simulink model "asghb"  (R2016a)
settings: Solver=VariableStepAuto  StartTime=0.0  StopTime=500  RelTol=1e-3
values from neighbouring files (symbols this model uses):
  Ag = 0.8    [Valori.m]
  Dg1 = 40    [Valori.m]
  Dg2 = 60    [Valori.m]
  Dg3 = 80    [Valori.m]
  Gb = 80    [Valori.m]
  K1 = 55.55    [Valori.m]
  K2 = 1260000    [Valori.m]
  K3 = 132.312    [Valori.m]
  n = 0.109    [Valori.m]
  p1 = 0.029    [Valori.m]
  p2 = 0.029    [Valori.m]
  p3 = 0.00000783    (= 7.83e-06)    [Valori.m]
  tgmax = 40    [Valori.m]
  V = 120    [Valori.m]
settings Model: Creator=carme  LastModifiedBy=carme

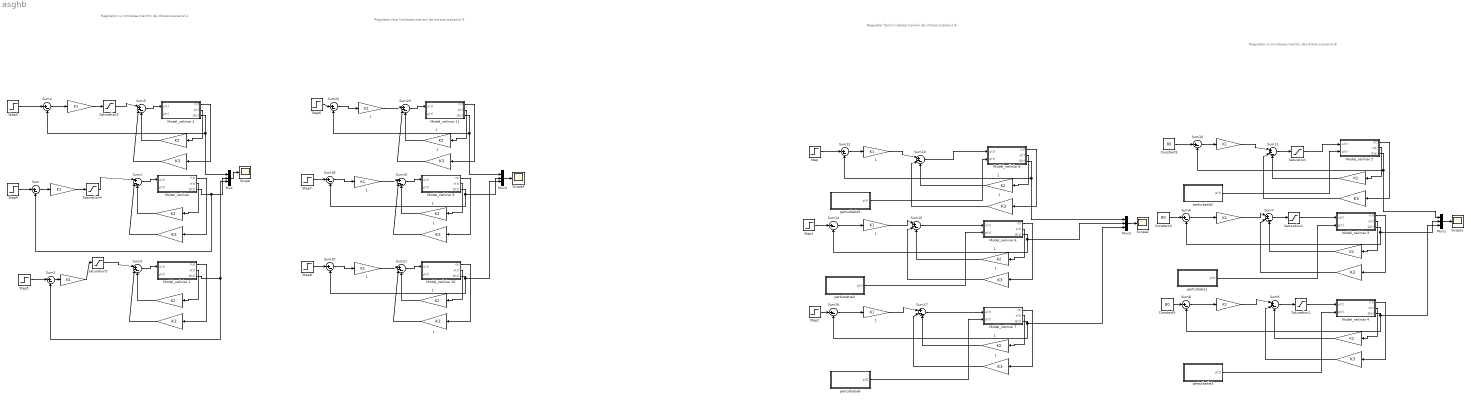
== system asghb ==
  note: Regulator cu limitarea marimii de intrare scenariul A
  note: Regulator cu limitarea marimii de intrare scenariul B
  note: Regulator fara limitarea marimii de intrare scenariul B
  note: Regulator fara limitarea marimii de intrare scenariul A
   {,,1,1} (4 alike) : Gain  Gain=K1
  "   " : Gain  Gain=K3
  "      " : Gain  Gain=K3
  "       " : Gain  Gain=K2
  "        " : Gain  Gain=K2
  "          " : Gain  Gain=K3
  "              " : Gain  Gain=K2
  "               " : Gain  Gain=K1
  " " : Gain  Gain=K2
  " 1" : Gain  Gain=K2
  "                                  " : Gain  Gain=K3
  "                                        " : Gain  Gain=K1
  "                                           " : Gain  Gain=K1
  "                                            " : Gain  Gain=K3
  "                                                        " : Gain  Gain=K1
  "                                                             " : Gain  Gain=K3
  "                                                                     " : Gain  Gain=K2
  "                                                                                           " : Gain  Gain=K2
  "                                                                                           1" : Gain  Gain=K2
  "                                                                     1" : Gain  Gain=K2
  "                                                             1" : Gain  Gain=K3
  "                                                        1" : Gain  Gain=K1
  "                                            1" : Gain  Gain=K3
  "                                           1" : Gain  Gain=K1
  "                                        1" : Gain  Gain=K1
  "                                  1" : Gain  Gain=K3
  "               1" : Gain  Gain=K1
  "              1" : Gain  Gain=K2
  "          1" : Gain  Gain=K3
  "        1" : Gain  Gain=K2
  "       1" : Gain  Gain=K2
  "      1" : Gain  Gain=K3
  "   1" : Gain  Gain=K3
  Constant3 : Constant  Value=80
  Constant4 : Constant  Value=80
  Constant5 : Constant  Value=80
  "Model_neliniar " : Subsystem
  Model_neliniar 1 : Subsystem
  Model_neliniar 10 : Subsystem
  Model_neliniar 11 : Subsystem
  Model_neliniar 2 : Subsystem
  Model_neliniar 3 : Subsystem
  Model_neliniar 4 : Subsystem
  Model_neliniar 5 : Subsystem
  Model_neliniar 6 : Subsystem
  Model_neliniar 7 : Subsystem
  Model_neliniar 8 : Subsystem
  Model_neliniar 9 : Subsystem
  Mux{,1..3} (4 alike) : Mux  Inputs=3
  Saturation{,1..5} (6 alike) : Saturate
  Scope{,1..3} (4 alike) : Scope
  Step{,1..8} (9 alike) : Step  SampleTime=0
  Sum{,2,4,6,8,10,12,14,16,18,20,22} (12 alike) : Sum  Inputs=|+-
  Sum{1,3,5,7,9,11,13,15,17,19,21,23} (12 alike) : Sum  Inputs=|+--
  perturbatie1 : Subsystem
  perturbatie2 : Subsystem
  perturbatie3 : Subsystem
  perturbatie4 : Subsystem
  perturbatie5 : Subsystem
  perturbatie6 : Subsystem
  wires:
  Sum1/1 -> "Model_neliniar "/1(u(t))
  "Model_neliniar "/3(G(t)) -> Mux/2, Sum/2
  "Model_neliniar "/1(i(t)) -> "                                  "/1
  "Model_neliniar "/2(x(t)) -> "                                                                     "/1
  "                                  "/1 -> Sum1/2
  "                                                                     "/1 -> Sum1/3
  Step4/1 -> Sum/1
  Sum/1 -> "                                                        "/1
  Sum3/1 -> Model_neliniar 1/1(u(t))
  Model_neliniar 1/3(G(t)) -> Mux/3, Sum2/2
  Model_neliniar 1/1(i(t)) -> "                                                             "/1
  Model_neliniar 1/2(x(t)) -> "                                                                                           "/1
  "                                                             "/1 -> Sum3/2
  "                                                                                           "/1 -> Sum3/3
  Step5/1 -> Sum2/1
  Sum2/1 -> "                                        "/1
  Sum5/1 -> Model_neliniar 2/1(u(t))
  Model_neliniar 2/3(G(t)) -> Mux/1, Sum4/2
  Model_neliniar 2/1(i(t)) -> "                                            "/1
  Model_neliniar 2/2(x(t)) -> "              "/1
  "                                            "/1 -> Sum5/2
  "              "/1 -> Sum5/3
  Step3/1 -> Sum4/1
  Sum4/1 -> " "/1
  Mux/1 -> Scope/1
  "               "/1 -> Sum7/1
  Model_neliniar 3/3(G(t)) -> Mux1/2, Sum6/2
  Model_neliniar 3/1(i(t)) -> "      "/1
  Model_neliniar 3/2(x(t)) -> "        "/1
  "      "/1 -> Sum7/2
  "        "/1 -> Sum7/3
  Constant4/1 -> Sum6/1
  Sum6/1 -> "               "/1
  "                                           "/1 -> Sum9/1
  Model_neliniar 4/3(G(t)) -> Mux1/3, Sum8/2
  Model_neliniar 4/1(i(t)) -> "   "/1
  Model_neliniar 4/2(x(t)) -> "       "/1
  "   "/1 -> Sum9/2
  "       "/1 -> Sum9/3
  Constant5/1 -> Sum8/1
  Sum8/1 -> "                                           "/1
  " "/1 -> Sum11/1
  Model_neliniar 5/3(G(t)) -> Mux1/1, Sum10/2
  Model_neliniar 5/1(i(t)) -> "          "/1
  Model_neliniar 5/2(x(t)) -> " "/1
  "          "/1 -> Sum11/2
  " "/1 -> Sum11/3
  Constant3/1 -> Sum10/1
  Sum10/1 -> " "/1
  Mux1/1 -> Scope1/1
  Sum11/1 -> Saturation/1
  Saturation/1 -> Model_neliniar 5/1(u(t))
  Sum7/1 -> Saturation1/1
  Saturation1/1 -> Model_neliniar 3/1(u(t))
  Sum9/1 -> Saturation2/1
  Saturation2/1 -> Model_neliniar 4/1(u(t))
  perturbatie2/1(p(t)) -> Model_neliniar 5/2(p(t))
  perturbatie1/1(p(t)) -> Model_neliniar 3/2(p(t))
  perturbatie3/1(p(t)) -> Model_neliniar 4/2(p(t))
  "               1"/1 -> Sum15/1
  Model_neliniar 6/3(G(t)) -> Mux2/2, Sum14/2
  Model_neliniar 6/1(i(t)) -> "      1"/1
  Model_neliniar 6/2(x(t)) -> "        1"/1
  "      1"/1 -> Sum15/2
  "        1"/1 -> Sum15/3
  Step1/1 -> Sum14/1
  Sum14/1 -> "               1"/1
  "                                           1"/1 -> Sum17/1
  Model_neliniar 7/3(G(t)) -> Mux2/3, Sum16/2
  Model_neliniar 7/1(i(t)) -> "   1"/1
  Model_neliniar 7/2(x(t)) -> "       1"/1
  "   1"/1 -> Sum17/2
  "       1"/1 -> Sum17/3
  Step2/1 -> Sum16/1
  Sum16/1 -> "                                           1"/1
  " 1"/1 -> Sum13/1
  Model_neliniar 8/3(G(t)) -> Mux2/1, Sum12/2
  Model_neliniar 8/1(i(t)) -> "          1"/1
  Model_neliniar 8/2(x(t)) -> " 1"/1
  "          1"/1 -> Sum13/2
  " 1"/1 -> Sum13/3
  Step/1 -> Sum12/1
  Sum12/1 -> " 1"/1
  Mux2/1 -> Scope2/1
  Sum13/1 -> Model_neliniar 8/1(u(t))
  Sum15/1 -> Model_neliniar 6/1(u(t))
  Sum17/1 -> Model_neliniar 7/1(u(t))
  perturbatie5/1(p(t)) -> Model_neliniar 8/2(p(t))
  perturbatie4/1(p(t)) -> Model_neliniar 6/2(p(t))
  perturbatie6/1(p(t)) -> Model_neliniar 7/2(p(t))
  "                                                        1"/1 -> Sum19/1
  Sum19/1 -> Model_neliniar 9/1(u(t))
  Model_neliniar 9/3(G(t)) -> Mux3/2, Sum18/2
  Model_neliniar 9/1(i(t)) -> "                                  1"/1
  Model_neliniar 9/2(x(t)) -> "                                                                     1"/1
  "                                  1"/1 -> Sum19/2
  "                                                                     1"/1 -> Sum19/3
  Step7/1 -> Sum18/1
  Sum18/1 -> "                                                        1"/1
  "                                        1"/1 -> Sum21/1
  Sum21/1 -> Model_neliniar 10/1(u(t))
  Model_neliniar 10/3(G(t)) -> Mux3/3, Sum20/2
  Model_neliniar 10/1(i(t)) -> "                                                             1"/1
  Model_neliniar 10/2(x(t)) -> "                                                                                           1"/1
  "                                                             1"/1 -> Sum21/2
  "                                                                                           1"/1 -> Sum21/3
  Step8/1 -> Sum20/1
  Sum20/1 -> "                                        1"/1
  " 1"/1 -> Sum23/1
  Sum23/1 -> Model_neliniar 11/1(u(t))
  Model_neliniar 11/3(G(t)) -> Mux3/1, Sum22/2
  Model_neliniar 11/1(i(t)) -> "                                            1"/1
  Model_neliniar 11/2(x(t)) -> "              1"/1
  "                                            1"/1 -> Sum23/2
  "              1"/1 -> Sum23/3
  Step6/1 -> Sum22/1
  Sum22/1 -> " 1"/1
  Mux3/1 -> Scope3/1
  " "/1 -> Saturation3/1
  Saturation3/1 -> Sum5/1
  "                                                        "/1 -> Saturation4/1
  Saturation4/1 -> Sum1/1
  "                                        "/1 -> Saturation5/1
  Saturation5/1 -> Sum3/1

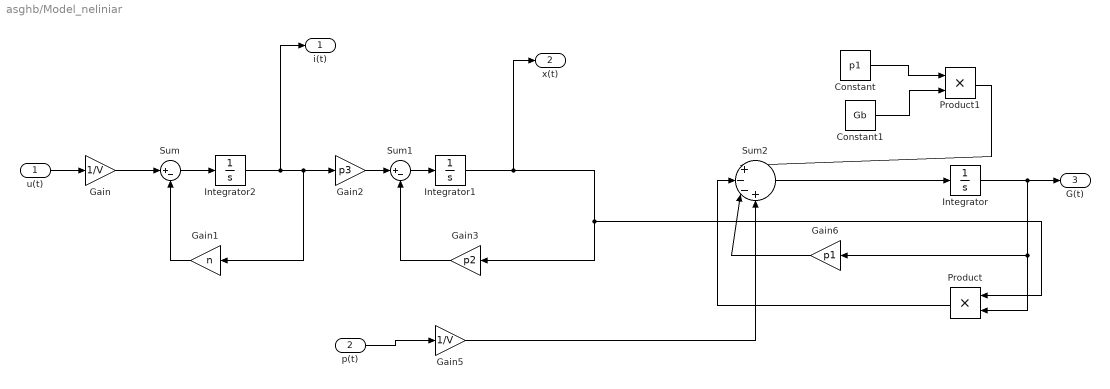
== system asghb/Model_neliniar  ==
  u(t) : Inport
  p(t) : Inport  Port=2
  Constant : Constant  Value=p1
  Constant1 : Constant  Value=Gb
  Gain : Gain  Gain=1/V
  Gain1 : Gain  Gain=n
  Gain2 : Gain  Gain=p3
  Gain3 : Gain  Gain=p2
  Gain5 : Gain  Gain=1/V
  Gain6 : Gain  Gain=p1
  Integrator : Integrator  InitialCondition=200
  Integrator1 : Integrator
  Integrator2 : Integrator
  Product : Product
  Product1 : Product
  Sum : Sum  Inputs=|+-
  Sum1 : Sum  Inputs=|+-
  Sum2 : Sum  Inputs=|+--+
  i(t) : Outport
  x(t) : Outport  Port=2
  G(t) : Outport  Port=3
  wires:
  u(t)/1 -> Gain/1
  Gain/1 -> Sum/1
  Sum/1 -> Integrator2/1
  Integrator2/1 -> i(t)/1, Gain1/1, Gain2/1
  Gain2/1 -> Sum1/1
  Sum1/1 -> Integrator1/1
  Gain1/1 -> Sum/2
  Gain3/1 -> Sum1/2
  Integrator1/1 -> x(t)/1, Product/1, Gain3/1
  p(t)/1 -> Gain5/1
  Gain5/1 -> Sum2/4
  Integrator/1 -> Product/2, Gain6/1, G(t)/1
  Gain6/1 -> Sum2/3
  Constant/1 -> Product1/1
  Constant1/1 -> Product1/2
  Product1/1 -> Sum2/1
  Product/1 -> Sum2/2
  Sum2/1 -> Integrator/1

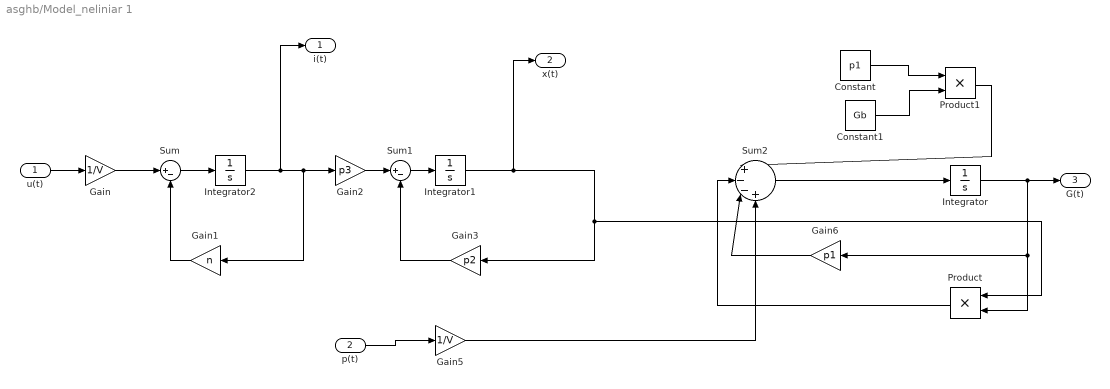
== system asghb/Model_neliniar 1 ==
  u(t) : Inport
  p(t) : Inport  Port=2
  Constant : Constant  Value=p1
  Constant1 : Constant  Value=Gb
  Gain : Gain  Gain=1/V
  Gain1 : Gain  Gain=n
  Gain2 : Gain  Gain=p3
  Gain3 : Gain  Gain=p2
  Gain5 : Gain  Gain=1/V
  Gain6 : Gain  Gain=p1
  Integrator : Integrator  InitialCondition=300
  Integrator1 : Integrator
  Integrator2 : Integrator
  Product : Product
  Product1 : Product
  Sum : Sum  Inputs=|+-
  Sum1 : Sum  Inputs=|+-
  Sum2 : Sum  Inputs=|+--+
  i(t) : Outport
  x(t) : Outport  Port=2
  G(t) : Outport  Port=3
  wires:
  u(t)/1 -> Gain/1
  Gain/1 -> Sum/1
  Sum/1 -> Integrator2/1
  Integrator2/1 -> i(t)/1, Gain1/1, Gain2/1
  Gain2/1 -> Sum1/1
  Sum1/1 -> Integrator1/1
  Gain1/1 -> Sum/2
  Gain3/1 -> Sum1/2
  Integrator1/1 -> x(t)/1, Product/1, Gain3/1
  p(t)/1 -> Gain5/1
  Gain5/1 -> Sum2/4
  Integrator/1 -> Product/2, Gain6/1, G(t)/1
  Gain6/1 -> Sum2/3
  Constant/1 -> Product1/1
  Constant1/1 -> Product1/2
  Product1/1 -> Sum2/1
  Product/1 -> Sum2/2
  Sum2/1 -> Integrator/1

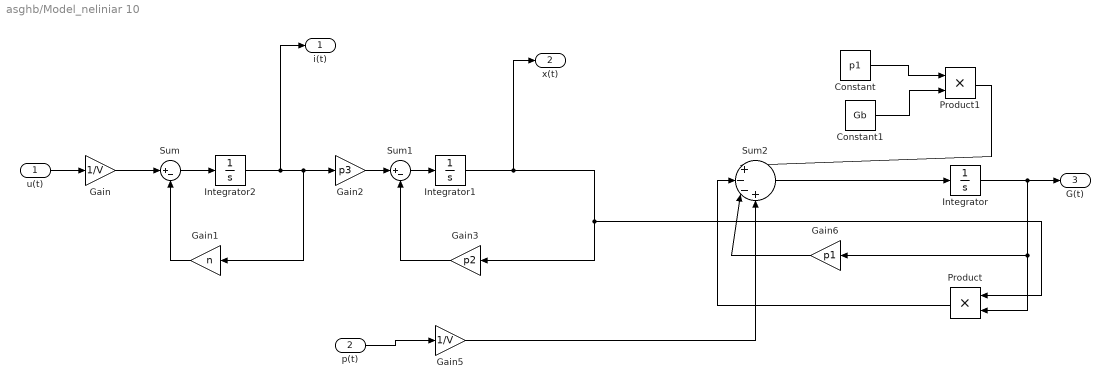
== system asghb/Model_neliniar 10 ==
  u(t) : Inport
  p(t) : Inport  Port=2
  Constant : Constant  Value=p1
  Constant1 : Constant  Value=Gb
  Gain : Gain  Gain=1/V
  Gain1 : Gain  Gain=n
  Gain2 : Gain  Gain=p3
  Gain3 : Gain  Gain=p2
  Gain5 : Gain  Gain=1/V
  Gain6 : Gain  Gain=p1
  Integrator : Integrator  InitialCondition=300
  Integrator1 : Integrator
  Integrator2 : Integrator
  Product : Product
  Product1 : Product
  Sum : Sum  Inputs=|+-
  Sum1 : Sum  Inputs=|+-
  Sum2 : Sum  Inputs=|+--+
  i(t) : Outport
  x(t) : Outport  Port=2
  G(t) : Outport  Port=3
  wires:
  u(t)/1 -> Gain/1
  Gain/1 -> Sum/1
  Sum/1 -> Integrator2/1
  Integrator2/1 -> i(t)/1, Gain1/1, Gain2/1
  Gain2/1 -> Sum1/1
  Sum1/1 -> Integrator1/1
  Gain1/1 -> Sum/2
  Gain3/1 -> Sum1/2
  Integrator1/1 -> x(t)/1, Product/1, Gain3/1
  p(t)/1 -> Gain5/1
  Gain5/1 -> Sum2/4
  Integrator/1 -> Product/2, Gain6/1, G(t)/1
  Gain6/1 -> Sum2/3
  Constant/1 -> Product1/1
  Constant1/1 -> Product1/2
  Product1/1 -> Sum2/1
  Product/1 -> Sum2/2
  Sum2/1 -> Integrator/1

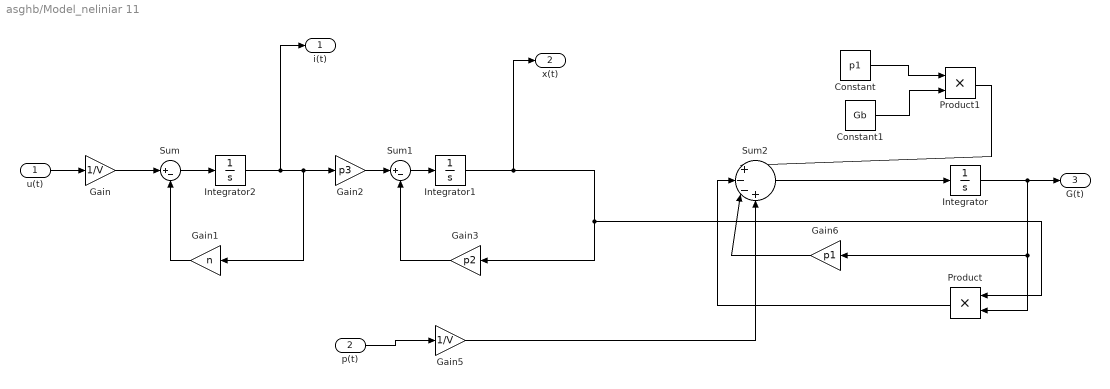
== system asghb/Model_neliniar 11 ==
  u(t) : Inport
  p(t) : Inport  Port=2
  Constant : Constant  Value=p1
  Constant1 : Constant  Value=Gb
  Gain : Gain  Gain=1/V
  Gain1 : Gain  Gain=n
  Gain2 : Gain  Gain=p3
  Gain3 : Gain  Gain=p2
  Gain5 : Gain  Gain=1/V
  Gain6 : Gain  Gain=p1
  Integrator : Integrator  InitialCondition=120
  Integrator1 : Integrator
  Integrator2 : Integrator
  Product : Product
  Product1 : Product
  Sum : Sum  Inputs=|+-
  Sum1 : Sum  Inputs=|+-
  Sum2 : Sum  Inputs=|+--+
  i(t) : Outport
  x(t) : Outport  Port=2
  G(t) : Outport  Port=3
  wires:
  u(t)/1 -> Gain/1
  Gain/1 -> Sum/1
  Sum/1 -> Integrator2/1
  Integrator2/1 -> i(t)/1, Gain1/1, Gain2/1
  Gain2/1 -> Sum1/1
  Sum1/1 -> Integrator1/1
  Gain1/1 -> Sum/2
  Gain3/1 -> Sum1/2
  Integrator1/1 -> x(t)/1, Product/1, Gain3/1
  p(t)/1 -> Gain5/1
  Gain5/1 -> Sum2/4
  Integrator/1 -> Product/2, Gain6/1, G(t)/1
  Gain6/1 -> Sum2/3
  Constant/1 -> Product1/1
  Constant1/1 -> Product1/2
  Product1/1 -> Sum2/1
  Product/1 -> Sum2/2
  Sum2/1 -> Integrator/1

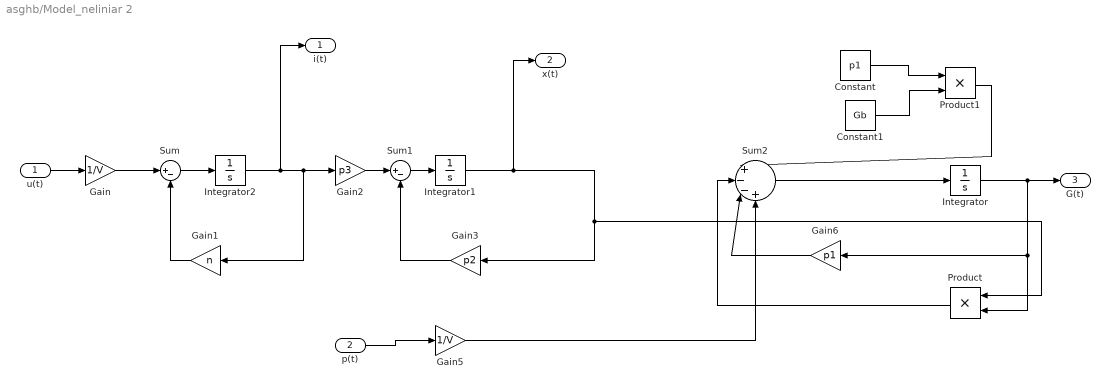
== system asghb/Model_neliniar 2 ==
  u(t) : Inport
  p(t) : Inport  Port=2
  Constant : Constant  Value=p1
  Constant1 : Constant  Value=Gb
  Gain : Gain  Gain=1/V
  Gain1 : Gain  Gain=n
  Gain2 : Gain  Gain=p3
  Gain3 : Gain  Gain=p2
  Gain5 : Gain  Gain=1/V
  Gain6 : Gain  Gain=p1
  Integrator : Integrator  InitialCondition=120
  Integrator1 : Integrator
  Integrator2 : Integrator
  Product : Product
  Product1 : Product
  Sum : Sum  Inputs=|+-
  Sum1 : Sum  Inputs=|+-
  Sum2 : Sum  Inputs=|+--+
  i(t) : Outport
  x(t) : Outport  Port=2
  G(t) : Outport  Port=3
  wires:
  u(t)/1 -> Gain/1
  Gain/1 -> Sum/1
  Sum/1 -> Integrator2/1
  Integrator2/1 -> i(t)/1, Gain1/1, Gain2/1
  Gain2/1 -> Sum1/1
  Sum1/1 -> Integrator1/1
  Gain1/1 -> Sum/2
  Gain3/1 -> Sum1/2
  Integrator1/1 -> x(t)/1, Product/1, Gain3/1
  p(t)/1 -> Gain5/1
  Gain5/1 -> Sum2/4
  Integrator/1 -> Product/2, Gain6/1, G(t)/1
  Gain6/1 -> Sum2/3
  Constant/1 -> Product1/1
  Constant1/1 -> Product1/2
  Product1/1 -> Sum2/1
  Product/1 -> Sum2/2
  Sum2/1 -> Integrator/1

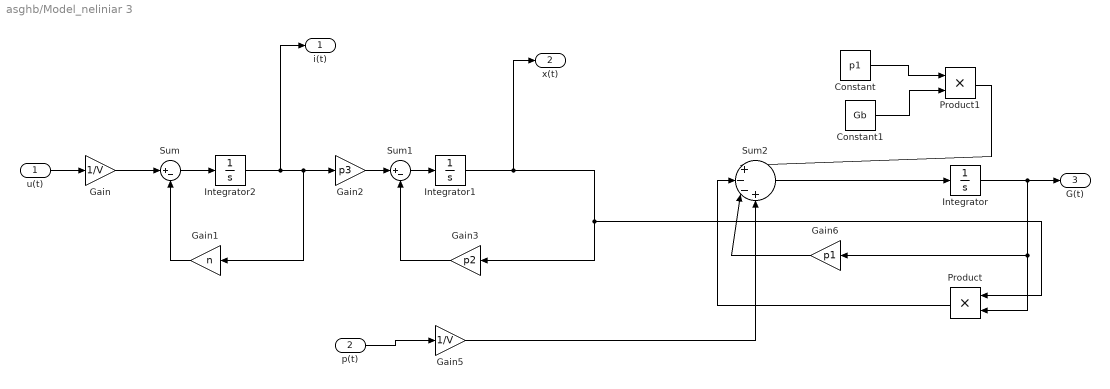
== system asghb/Model_neliniar 3 ==
  u(t) : Inport
  p(t) : Inport  Port=2
  Constant : Constant  Value=p1
  Constant1 : Constant  Value=Gb
  Gain : Gain  Gain=1/V
  Gain1 : Gain  Gain=n
  Gain2 : Gain  Gain=p3
  Gain3 : Gain  Gain=p2
  Gain5 : Gain  Gain=1/V
  Gain6 : Gain  Gain=p1
  Integrator : Integrator  InitialCondition=80
  Integrator1 : Integrator
  Integrator2 : Integrator
  Product : Product
  Product1 : Product
  Sum : Sum  Inputs=|+-
  Sum1 : Sum  Inputs=|+-
  Sum2 : Sum  Inputs=|+--+
  i(t) : Outport
  x(t) : Outport  Port=2
  G(t) : Outport  Port=3
  wires:
  u(t)/1 -> Gain/1
  Gain/1 -> Sum/1
  Sum/1 -> Integrator2/1
  Integrator2/1 -> i(t)/1, Gain1/1, Gain2/1
  Gain2/1 -> Sum1/1
  Sum1/1 -> Integrator1/1
  Gain1/1 -> Sum/2
  Gain3/1 -> Sum1/2
  Integrator1/1 -> x(t)/1, Product/1, Gain3/1
  p(t)/1 -> Gain5/1
  Gain5/1 -> Sum2/4
  Integrator/1 -> Product/2, Gain6/1, G(t)/1
  Gain6/1 -> Sum2/3
  Constant/1 -> Product1/1
  Constant1/1 -> Product1/2
  Product1/1 -> Sum2/1
  Product/1 -> Sum2/2
  Sum2/1 -> Integrator/1

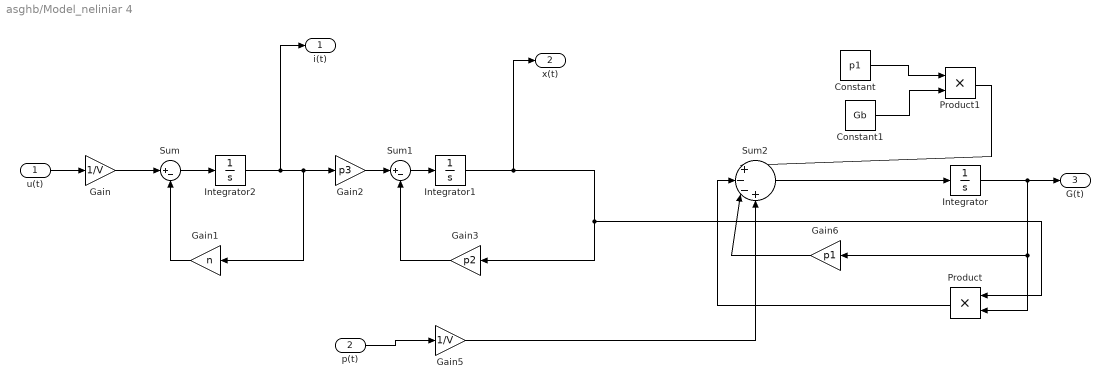
== system asghb/Model_neliniar 4 ==
  u(t) : Inport
  p(t) : Inport  Port=2
  Constant : Constant  Value=p1
  Constant1 : Constant  Value=Gb
  Gain : Gain  Gain=1/V
  Gain1 : Gain  Gain=n
  Gain2 : Gain  Gain=p3
  Gain3 : Gain  Gain=p2
  Gain5 : Gain  Gain=1/V
  Gain6 : Gain  Gain=p1
  Integrator : Integrator  InitialCondition=80
  Integrator1 : Integrator
  Integrator2 : Integrator
  Product : Product
  Product1 : Product
  Sum : Sum  Inputs=|+-
  Sum1 : Sum  Inputs=|+-
  Sum2 : Sum  Inputs=|+--+
  i(t) : Outport
  x(t) : Outport  Port=2
  G(t) : Outport  Port=3
  wires:
  u(t)/1 -> Gain/1
  Gain/1 -> Sum/1
  Sum/1 -> Integrator2/1
  Integrator2/1 -> i(t)/1, Gain1/1, Gain2/1
  Gain2/1 -> Sum1/1
  Sum1/1 -> Integrator1/1
  Gain1/1 -> Sum/2
  Gain3/1 -> Sum1/2
  Integrator1/1 -> x(t)/1, Product/1, Gain3/1
  p(t)/1 -> Gain5/1
  Gain5/1 -> Sum2/4
  Integrator/1 -> Product/2, Gain6/1, G(t)/1
  Gain6/1 -> Sum2/3
  Constant/1 -> Product1/1
  Constant1/1 -> Product1/2
  Product1/1 -> Sum2/1
  Product/1 -> Sum2/2
  Sum2/1 -> Integrator/1

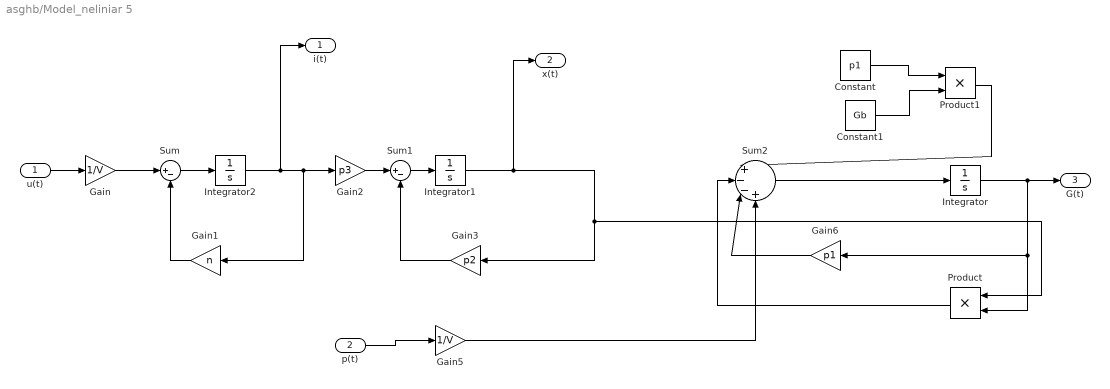
== system asghb/Model_neliniar 5 ==
  u(t) : Inport
  p(t) : Inport  Port=2
  Constant : Constant  Value=p1
  Constant1 : Constant  Value=Gb
  Gain : Gain  Gain=1/V
  Gain1 : Gain  Gain=n
  Gain2 : Gain  Gain=p3
  Gain3 : Gain  Gain=p2
  Gain5 : Gain  Gain=1/V
  Gain6 : Gain  Gain=p1
  Integrator : Integrator  InitialCondition=80
  Integrator1 : Integrator
  Integrator2 : Integrator
  Product : Product
  Product1 : Product
  Sum : Sum  Inputs=|+-
  Sum1 : Sum  Inputs=|+-
  Sum2 : Sum  Inputs=|+--+
  i(t) : Outport
  x(t) : Outport  Port=2
  G(t) : Outport  Port=3
  wires:
  u(t)/1 -> Gain/1
  Gain/1 -> Sum/1
  Sum/1 -> Integrator2/1
  Integrator2/1 -> i(t)/1, Gain1/1, Gain2/1
  Gain2/1 -> Sum1/1
  Sum1/1 -> Integrator1/1
  Gain1/1 -> Sum/2
  Gain3/1 -> Sum1/2
  Integrator1/1 -> x(t)/1, Product/1, Gain3/1
  p(t)/1 -> Gain5/1
  Gain5/1 -> Sum2/4
  Integrator/1 -> Product/2, Gain6/1, G(t)/1
  Gain6/1 -> Sum2/3
  Constant/1 -> Product1/1
  Constant1/1 -> Product1/2
  Product1/1 -> Sum2/1
  Product/1 -> Sum2/2
  Sum2/1 -> Integrator/1

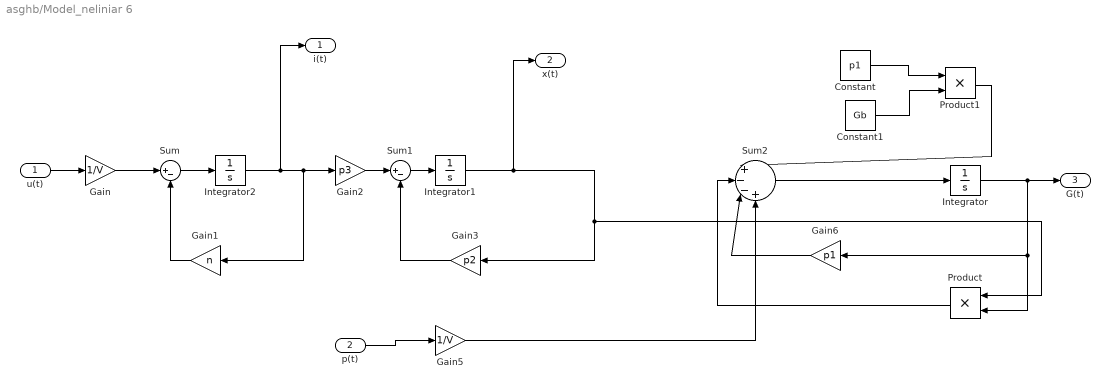
== system asghb/Model_neliniar 6 ==
  u(t) : Inport
  p(t) : Inport  Port=2
  Constant : Constant  Value=p1
  Constant1 : Constant  Value=Gb
  Gain : Gain  Gain=1/V
  Gain1 : Gain  Gain=n
  Gain2 : Gain  Gain=p3
  Gain3 : Gain  Gain=p2
  Gain5 : Gain  Gain=1/V
  Gain6 : Gain  Gain=p1
  Integrator : Integrator  InitialCondition=80
  Integrator1 : Integrator
  Integrator2 : Integrator
  Product : Product
  Product1 : Product
  Sum : Sum  Inputs=|+-
  Sum1 : Sum  Inputs=|+-
  Sum2 : Sum  Inputs=|+--+
  i(t) : Outport
  x(t) : Outport  Port=2
  G(t) : Outport  Port=3
  wires:
  u(t)/1 -> Gain/1
  Gain/1 -> Sum/1
  Sum/1 -> Integrator2/1
  Integrator2/1 -> i(t)/1, Gain1/1, Gain2/1
  Gain2/1 -> Sum1/1
  Sum1/1 -> Integrator1/1
  Gain1/1 -> Sum/2
  Gain3/1 -> Sum1/2
  Integrator1/1 -> x(t)/1, Product/1, Gain3/1
  p(t)/1 -> Gain5/1
  Gain5/1 -> Sum2/4
  Integrator/1 -> Product/2, Gain6/1, G(t)/1
  Gain6/1 -> Sum2/3
  Constant/1 -> Product1/1
  Constant1/1 -> Product1/2
  Product1/1 -> Sum2/1
  Product/1 -> Sum2/2
  Sum2/1 -> Integrator/1

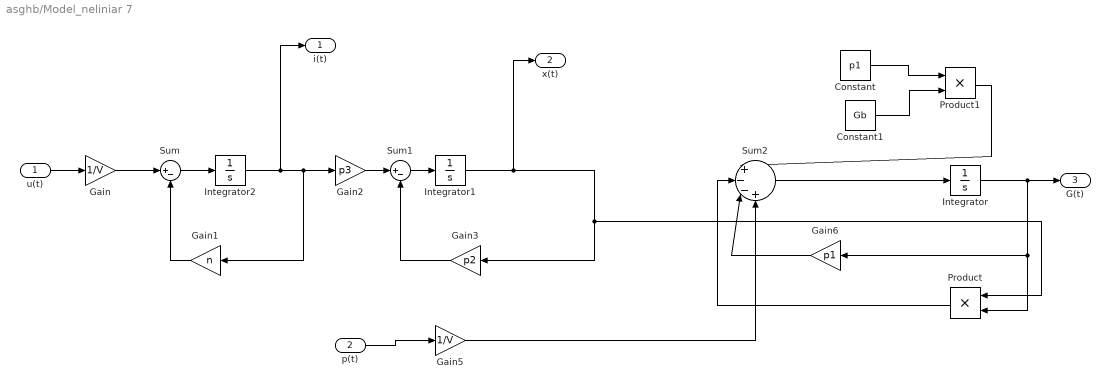
== system asghb/Model_neliniar 7 ==
  u(t) : Inport
  p(t) : Inport  Port=2
  Constant : Constant  Value=p1
  Constant1 : Constant  Value=Gb
  Gain : Gain  Gain=1/V
  Gain1 : Gain  Gain=n
  Gain2 : Gain  Gain=p3
  Gain3 : Gain  Gain=p2
  Gain5 : Gain  Gain=1/V
  Gain6 : Gain  Gain=p1
  Integrator : Integrator  InitialCondition=80
  Integrator1 : Integrator
  Integrator2 : Integrator
  Product : Product
  Product1 : Product
  Sum : Sum  Inputs=|+-
  Sum1 : Sum  Inputs=|+-
  Sum2 : Sum  Inputs=|+--+
  i(t) : Outport
  x(t) : Outport  Port=2
  G(t) : Outport  Port=3
  wires:
  u(t)/1 -> Gain/1
  Gain/1 -> Sum/1
  Sum/1 -> Integrator2/1
  Integrator2/1 -> i(t)/1, Gain1/1, Gain2/1
  Gain2/1 -> Sum1/1
  Sum1/1 -> Integrator1/1
  Gain1/1 -> Sum/2
  Gain3/1 -> Sum1/2
  Integrator1/1 -> x(t)/1, Product/1, Gain3/1
  p(t)/1 -> Gain5/1
  Gain5/1 -> Sum2/4
  Integrator/1 -> Product/2, Gain6/1, G(t)/1
  Gain6/1 -> Sum2/3
  Constant/1 -> Product1/1
  Constant1/1 -> Product1/2
  Product1/1 -> Sum2/1
  Product/1 -> Sum2/2
  Sum2/1 -> Integrator/1

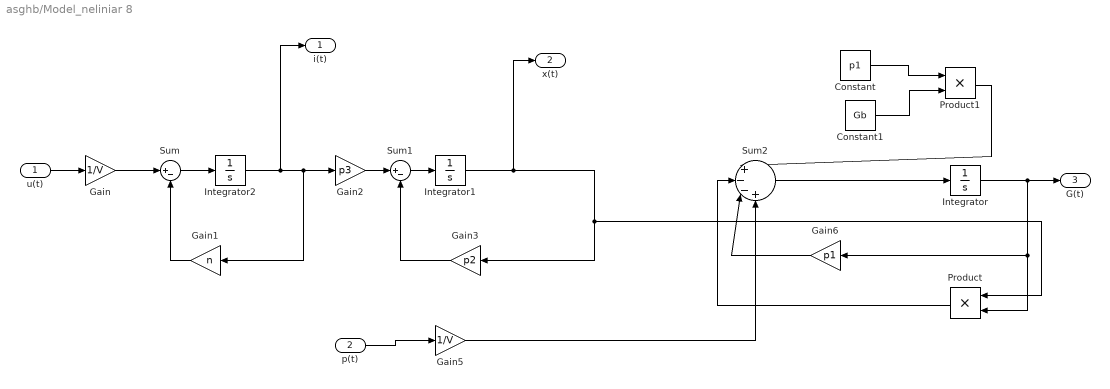
== system asghb/Model_neliniar 8 ==
  u(t) : Inport
  p(t) : Inport  Port=2
  Constant : Constant  Value=p1
  Constant1 : Constant  Value=Gb
  Gain : Gain  Gain=1/V
  Gain1 : Gain  Gain=n
  Gain2 : Gain  Gain=p3
  Gain3 : Gain  Gain=p2
  Gain5 : Gain  Gain=1/V
  Gain6 : Gain  Gain=p1
  Integrator : Integrator  InitialCondition=80
  Integrator1 : Integrator
  Integrator2 : Integrator
  Product : Product
  Product1 : Product
  Sum : Sum  Inputs=|+-
  Sum1 : Sum  Inputs=|+-
  Sum2 : Sum  Inputs=|+--+
  i(t) : Outport
  x(t) : Outport  Port=2
  G(t) : Outport  Port=3
  wires:
  u(t)/1 -> Gain/1
  Gain/1 -> Sum/1
  Sum/1 -> Integrator2/1
  Integrator2/1 -> i(t)/1, Gain1/1, Gain2/1
  Gain2/1 -> Sum1/1
  Sum1/1 -> Integrator1/1
  Gain1/1 -> Sum/2
  Gain3/1 -> Sum1/2
  Integrator1/1 -> x(t)/1, Product/1, Gain3/1
  p(t)/1 -> Gain5/1
  Gain5/1 -> Sum2/4
  Integrator/1 -> Product/2, Gain6/1, G(t)/1
  Gain6/1 -> Sum2/3
  Constant/1 -> Product1/1
  Constant1/1 -> Product1/2
  Product1/1 -> Sum2/1
  Product/1 -> Sum2/2
  Sum2/1 -> Integrator/1

== system asghb/Model_neliniar 9 ==
  u(t) : Inport
  p(t) : Inport  Port=2
  Constant : Constant  Value=p1
  Constant1 : Constant  Value=Gb
  Gain : Gain  Gain=1/V
  Gain1 : Gain  Gain=n
  Gain2 : Gain  Gain=p3
  Gain3 : Gain  Gain=p2
  Gain5 : Gain  Gain=1/V
  Gain6 : Gain  Gain=p1
  Integrator : Integrator  InitialCondition=200
  Integrator1 : Integrator
  Integrator2 : Integrator
  Product : Product
  Product1 : Product
  Sum : Sum  Inputs=|+-
  Sum1 : Sum  Inputs=|+-
  Sum2 : Sum  Inputs=|+--+
  i(t) : Outport
  x(t) : Outport  Port=2
  G(t) : Outport  Port=3
  wires:
  u(t)/1 -> Gain/1
  Gain/1 -> Sum/1
  Sum/1 -> Integrator2/1
  Integrator2/1 -> i(t)/1, Gain1/1, Gain2/1
  Gain2/1 -> Sum1/1
  Sum1/1 -> Integrator1/1
  Gain1/1 -> Sum/2
  Gain3/1 -> Sum1/2
  Integrator1/1 -> x(t)/1, Product/1, Gain3/1
  p(t)/1 -> Gain5/1
  Gain5/1 -> Sum2/4
  Integrator/1 -> Product/2, Gain6/1, G(t)/1
  Gain6/1 -> Sum2/3
  Constant/1 -> Product1/1
  Constant1/1 -> Product1/2
  Product1/1 -> Sum2/1
  Product/1 -> Sum2/2
  Sum2/1 -> Integrator/1

== system asghb/perturbatie1 ==
  Ag : Constant  Value=Ag
  "Clock " : Clock
  Dg : Constant  Value=Dg2
  Divide : Product  Inputs=*/
  Divide1 : Product  Inputs=*/
  Gain : Gain  Gain=-1
  Math Function : Math  SaturateOnIntegerOverflow=on
  Product : Product  Inputs=4
  Product1 : Product
  tg,max : Constant  Value=tgmax
  p(t) : Outport
  wires:
  Dg/1 -> Product/1
  Ag/1 -> Product/2
  Math Function/1 -> Product/3
  "Clock "/1 -> Product/4, Gain/1
  tg,max/1 -> Divide/2, Product1/2, Product1/1
  Divide/1 -> Math Function/1
  Gain/1 -> Divide/1
  Product1/1 -> Divide1/2
  Divide1/1 -> p(t)/1
  Product/1 -> Divide1/1

== system asghb/perturbatie2 ==
  Ag : Constant  Value=Ag
  "Clock " : Clock
  Dg : Constant  Value=Dg1
  Divide : Product  Inputs=*/
  Divide1 : Product  Inputs=*/
  Gain : Gain  Gain=-1
  Math Function : Math  SaturateOnIntegerOverflow=on
  Product : Product  Inputs=4
  Product1 : Product
  tg,max : Constant  Value=tgmax
  p(t) : Outport
  wires:
  Dg/1 -> Product/1
  Ag/1 -> Product/2
  Math Function/1 -> Product/3
  "Clock "/1 -> Product/4, Gain/1
  tg,max/1 -> Divide/2, Product1/2, Product1/1
  Divide/1 -> Math Function/1
  Gain/1 -> Divide/1
  Product1/1 -> Divide1/2
  Divide1/1 -> p(t)/1
  Product/1 -> Divide1/1

== system asghb/perturbatie3 ==
  Ag : Constant  Value=Ag
  "Clock " : Clock
  Dg : Constant  Value=Dg3
  Divide : Product  Inputs=*/
  Divide1 : Product  Inputs=*/
  Gain : Gain  Gain=-1
  Math Function : Math  SaturateOnIntegerOverflow=on
  Product : Product  Inputs=4
  Product1 : Product
  tg,max : Constant  Value=tgmax
  p(t) : Outport
  wires:
  Dg/1 -> Product/1
  Ag/1 -> Product/2
  Math Function/1 -> Product/3
  "Clock "/1 -> Product/4, Gain/1
  tg,max/1 -> Divide/2, Product1/2, Product1/1
  Divide/1 -> Math Function/1
  Gain/1 -> Divide/1
  Product1/1 -> Divide1/2
  Divide1/1 -> p(t)/1
  Product/1 -> Divide1/1

== system asghb/perturbatie4 ==
  Ag : Constant  Value=Ag
  "Clock " : Clock
  Dg : Constant  Value=Dg2
  Divide : Product  Inputs=*/
  Divide1 : Product  Inputs=*/
  Gain : Gain  Gain=-1
  Math Function : Math  SaturateOnIntegerOverflow=on
  Product : Product  Inputs=4
  Product1 : Product
  tg,max : Constant  Value=tgmax
  p(t) : Outport
  wires:
  Dg/1 -> Product/1
  Ag/1 -> Product/2
  Math Function/1 -> Product/3
  "Clock "/1 -> Product/4, Gain/1
  tg,max/1 -> Divide/2, Product1/2, Product1/1
  Divide/1 -> Math Function/1
  Gain/1 -> Divide/1
  Product1/1 -> Divide1/2
  Divide1/1 -> p(t)/1
  Product/1 -> Divide1/1

== system asghb/perturbatie5 ==
  Ag : Constant  Value=Ag
  "Clock " : Clock
  Dg : Constant  Value=Dg1
  Divide : Product  Inputs=*/
  Divide1 : Product  Inputs=*/
  Gain : Gain  Gain=-1
  Math Function : Math  SaturateOnIntegerOverflow=on
  Product : Product  Inputs=4
  Product1 : Product
  tg,max : Constant  Value=tgmax
  p(t) : Outport
  wires:
  Dg/1 -> Product/1
  Ag/1 -> Product/2
  Math Function/1 -> Product/3
  "Clock "/1 -> Product/4, Gain/1
  tg,max/1 -> Divide/2, Product1/2, Product1/1
  Divide/1 -> Math Function/1
  Gain/1 -> Divide/1
  Product1/1 -> Divide1/2
  Divide1/1 -> p(t)/1
  Product/1 -> Divide1/1

== system asghb/perturbatie6 ==
  Ag : Constant  Value=Ag
  "Clock " : Clock
  Dg : Constant  Value=Dg3
  Divide : Product  Inputs=*/
  Divide1 : Product  Inputs=*/
  Gain : Gain  Gain=-1
  Math Function : Math  SaturateOnIntegerOverflow=on
  Product : Product  Inputs=4
  Product1 : Product
  tg,max : Constant  Value=tgmax
  p(t) : Outport
  wires:
  Dg/1 -> Product/1
  Ag/1 -> Product/2
  Math Function/1 -> Product/3
  "Clock "/1 -> Product/4, Gain/1
  tg,max/1 -> Divide/2, Product1/2, Product1/1
  Divide/1 -> Math Function/1
  Gain/1 -> Divide/1
  Product1/1 -> Divide1/2
  Divide1/1 -> p(t)/1
  Product/1 -> Divide1/1
